simulink model "etr_14b_arch_cleanup"  (R2014b)
settings: Solver=FixedStepDiscrete  SolverMode=SingleTasking  StartTime=0.0  StopTime=inf  FixedStep=balancer_ts  RelTol=1e-3
undefined symbols (not defined in the file): a_d, a_r, balancerStates_Bus0, Batt, battery_gain, battery_offset, cmd_max, current_mode_status, current_task_operation_status, exec_period, Init_Bus0, k_f, k_i, k_phidot, k_thetadot, lightCalib, phi_des, R, STATE, TRACK_MODE_LIST, ts2, W
libraries: legonxtlib x27, simulink x19, simulink_extras x4, ControllersFcns x3, NXTFcns x1
(part 1 of 4)
settings Model: DataDictionary=mainDict.sldd  ExtModeTrigDuration=2  Creator=mbiesiad  LastModifiedBy=pvinnako
settings ConfigSet: Description=Use this configuration to communicate between two robots. This robot is the master.
settings OptimizationCC: OptimizeModelRefInitCode=on  LifeSpan=1
settings DebuggingCC: SolverPrmCheckMsg=none  ParameterPrecisionLossMsg=none  SignalLabelMismatchMsg=error  NonBusSignalsTreatedAsBus=error
settings HardwareCC: ProdLargestAtomicInteger=Long  ProdLargestAtomicFloat=Float  ProdEndianess=LittleEndian  ProdHWDeviceType=ARM Compatible->ARM 7
settings RTWCC: SystemTargetFile=realtime.tlc  GenerateMakefile=off  TemplateMakefile=realtime.tmf  Description=Run on Target Hardware  RTWVerbose=off  ProcessScript=realtime_make_rtw_hook
settings STFCustomTargetCC: TargetLibSuffix=.a  GenerateSampleERTMain=on  ERTCustomFileBanners=on  SupportNonInlinedSFcns=off  SupportVariableSizeSignals=on  MATLABClassNameForMDSCustomization=Simulink.SoftwareTarget.ERTCustomization  GRTInterface=off  SystemTargetFile=realtime.tlc
settings ERTTargetCC: GenerateSampleERTMain=on  ParMdlRefBuildCompliant=off  CompOptLevelCompliant=off  ConcurrentExecutionCompliant=off  CombineOutputUpdateFcns=off  ERTFirstTimeCompliant=off  SupportContinuousTime=on  SupportVariableSizeSignals=on  ModelStepFunctionPrototypeControlCompliant=off  CPPClassGenCompliant=off  ExtModeTransport=1  ExtModeMexFile=ext_serial_win32_comm_no_acks_rtt_byteswap  ExtModeMexArgs=0 1 9600  InlinedParameterPlacement=NonHierarchical  ERTSrcFileBannerTemplate=realtime_code_template.cgt  ERTHdrFileBannerTemplate=realtime_code_template.cgt  ERTDataSrcFileTemplate=realtime_code_template.cgt  ERTDataHdrFileTemplate=realtime_code_template.cgt  ERTCustomFileTemplate=realtime_file_process.tlc

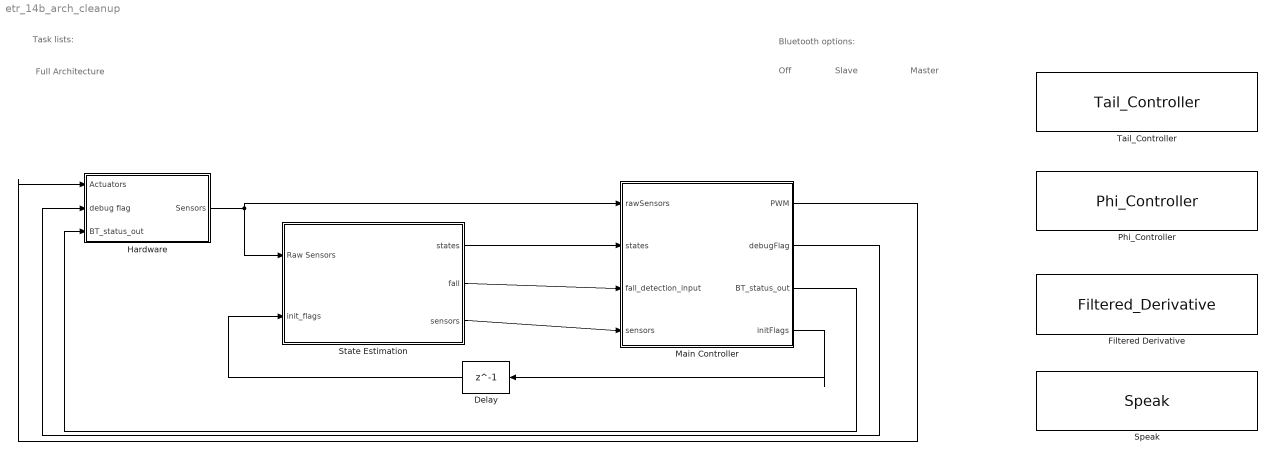
== system etr_14b_arch_cleanup ==
  note: Task lists:
  note: Bluetooth options:
  note: Slave
  note: Master
  note: Off
  note: Full Architecture
  Delay : Delay  DelayLength=1
  Filtered Derivative : ControllersFcns/Filtered_Derivative
  Hardware : Subsystem  VariantControl=Variant1
  Main Controller : Stateflow chart  TreatAsAtomicUnit=on
  Phi_Controller : ControllersFcns/Phi_Controller
  Speak : NXTFcns/Speak
  State Estimation : Subsystem
  Tail_Controller : ControllersFcns/Tail_Controller
  wires:
  State Estimation/2(fall) -> Main Controller/3(fall_detection_input)
  State Estimation/3(sensors) -> Main Controller/4(sensors)
  Hardware/1(Sensors) -> Main Controller/1(rawSensors), State Estimation/1(Raw Sensors)
  Main Controller/4(initFlags) -> Delay/1
  State Estimation/1(states) -> Main Controller/2(states)
  Delay/1 -> State Estimation/2(init_flags)
  Main Controller/2(debugFlag) -> Hardware/2(debug flag)
  Main Controller/1(PWM) -> Hardware/1(Actuators)
  Main Controller/3(BT_status_out) -> Hardware/3(BT_status_out)

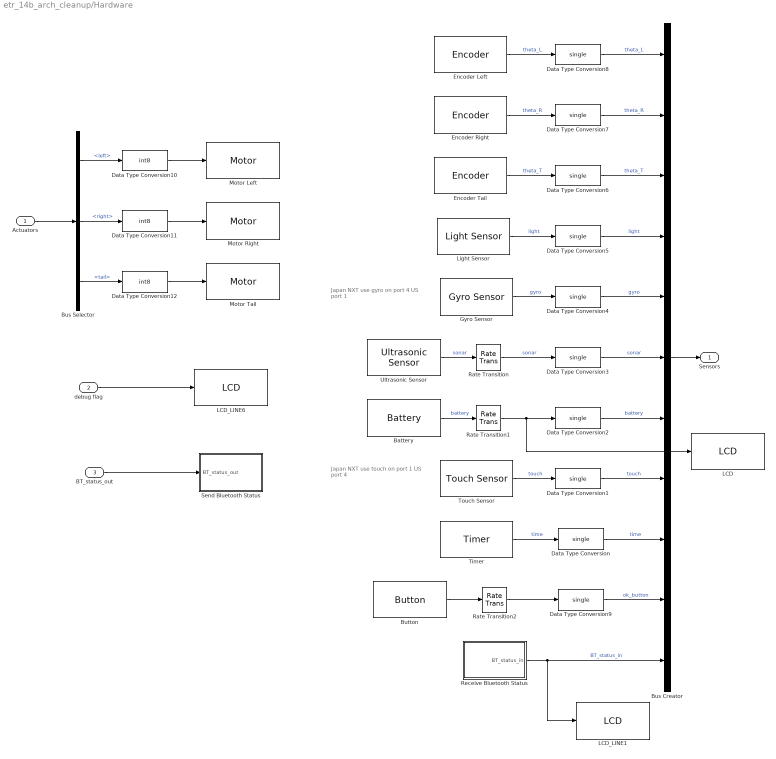
== system etr_14b_arch_cleanup/Hardware ==
  note: Japan NXT use gyro on port 4
      | US port 1
  note: Japan NXT use touch  on port 1
      | US port 4
  Actuators : Inport
  debug flag : Inport  Port=2
  BT_status_out : Inport  Port=3
  Battery : legonxtlib/Battery  sampleTime=.1
  Bus Creator : BusCreator  Inputs=11
  Bus Selector : BusSelector  OutputSignals=left,right,tail
  Button : legonxtlib/Button  buttonType=Middle orange  sampleTime=0.1
  Data Type Conversion{,1..9} (10 alike) : DataTypeConversion  OutDataTypeStr=single
  Data Type Conversion10 : DataTypeConversion  OutDataTypeStr=int8  SaturateOnIntegerOverflow=on
  Data Type Conversion11 : DataTypeConversion  OutDataTypeStr=int8  SaturateOnIntegerOverflow=on
  Data Type Conversion12 : DataTypeConversion  OutDataTypeStr=int8  SaturateOnIntegerOverflow=on
  Encoder Left : legonxtlib/Encoder  portNumber=C  opMode=No reset  sampleTime=0.004
  Encoder Right : legonxtlib/Encoder  portNumber=B  opMode=No reset  sampleTime=0.004
  Encoder Tail : legonxtlib/Encoder  portNumber=A  opMode=No reset  sampleTime=0.004
  Gyro Sensor : legonxtlib/Gyro Sensor  portNumber=1  outputMode=Raw A/D (0 - 1023)  offset=599  sampleTime=0.004
  LCD : legonxtlib/LCD  slcdStr=Batt:  slcdLine=3  slcdFormat=Decimal
  LCD_LINE1 : legonxtlib/LCD  slcdStr=BTSTAT  slcdLine=2  slcdFormat=Decimal
  LCD_LINE6 : legonxtlib/LCD  slcdStr=STATE:  slcdLine=1  slcdFormat=Decimal
  Light Sensor : legonxtlib/Light Sensor  portNumber=3  outputMode=Raw A/D (1023 - 0)  lightOn=on  sampleTime=0.004
  Motor Left : legonxtlib/Motor  sportNumber=C  sstopAction=Brake
  Motor Right : legonxtlib/Motor  sportNumber=B  sstopAction=Brake
  Motor Tail : legonxtlib/Motor  sportNumber=A  sstopAction=Brake
  Rate Transition : RateTransition  OutPortSampleTime=0.004
  Rate Transition1 : RateTransition  OutPortSampleTime=0.004
  Rate Transition2 : RateTransition  OutPortSampleTime=0.004
  Receive Bluetooth Status : Subsystem  Variant=on  OverrideUsingVariant=BluetoothOFF
  Send Bluetooth Status : Subsystem  Variant=on  OverrideUsingVariant=BluetoothOFF
  Timer : legonxtlib/Timer  sampleTime=0.004
  Touch Sensor : legonxtlib/Touch Sensor  portNumber=4  sampleTime=0.004
  Ultrasonic Sensor : legonxtlib/Ultrasonic Sensor  PortNumber=2  sampleTime=0.02
  Sensors : Outport
  wires:
  Receive Bluetooth Status/1(BT_status_in) -> LCD_LINE1/1, Bus Creator/11  "BT_status_in"
  debug flag/1 -> LCD_LINE6/1
  Data Type Conversion9/1 -> Bus Creator/10  "ok_button"
  Rate Transition2/1 -> Data Type Conversion9/1
  Button/1 -> Rate Transition2/1
  Rate Transition1/1 -> LCD/1, Data Type Conversion2/1
  Data Type Conversion8/1 -> Bus Creator/1  "theta_L"
  Data Type Conversion7/1 -> Bus Creator/2  "theta_R"
  Data Type Conversion6/1 -> Bus Creator/3  "theta_T"
  Data Type Conversion5/1 -> Bus Creator/4  "light"
  Data Type Conversion4/1 -> Bus Creator/5  "gyro"
  Data Type Conversion3/1 -> Bus Creator/6  "sonar"
  Data Type Conversion2/1 -> Bus Creator/7  "battery"
  Data Type Conversion1/1 -> Bus Creator/8  "touch"
  Data Type Conversion/1 -> Bus Creator/9  "time"
  Rate Transition/1 -> Data Type Conversion3/1  "sonar"
  Ultrasonic Sensor/1 -> Rate Transition/1  "sonar"
  Bus Selector/3 -> Data Type Conversion12/1  "<tail>"
  Encoder Tail/1 -> Data Type Conversion6/1  "theta_T"
  Light Sensor/1 -> Data Type Conversion5/1  "light"
  Bus Selector/2 -> Data Type Conversion11/1  "<right>"
  Bus Selector/1 -> Data Type Conversion10/1  "<left>"
  Touch Sensor/1 -> Data Type Conversion1/1  "touch"
  Bus Creator/1 -> Sensors/1
  Battery/1 -> Rate Transition1/1  "battery"
  Gyro Sensor/1 -> Data Type Conversion4/1  "gyro"
  Encoder Right/1 -> Data Type Conversion7/1  "theta_R"
  Encoder Left/1 -> Data Type Conversion8/1  "theta_L"
  Timer/1 -> Data Type Conversion/1  "time"
  Actuators/1 -> Bus Selector/1
  Data Type Conversion10/1 -> Motor Left/1
  Data Type Conversion11/1 -> Motor Right/1
  Data Type Conversion12/1 -> Motor Tail/1
  BT_status_out/1 -> Send Bluetooth Status/1(BT_status_out)

== system etr_14b_arch_cleanup/Main Controller/normal_operation_modes.gyro_calibration_mode ==
  sensors : Inport
  " Demux " : Demux  Outputs=1
  " SFunction " : S-Function  Tag=Stateflow S-Function etr_14b_arch_cleanup 10  FunctionName=sf_sfun  PortCounts=[1 4]  EnableBusSupport=off
  gyro_calibration_mode.GyroCalibration.Speak : Subsystem  Commented=on
      settings: UndoDeleteFcn=Stateflow.SLINSF.SimulinkMan.restorePreDeleteFcn  PreDeleteFcn=Stateflow.SLINSF.SimulinkMan.removePreDeleteFcn
  debugFlag : Outport
  initFlags : Outport  Port=2
  PWM : Outport  Port=3
  wires:
  sensors/1 -> " SFunction "/1
  " SFunction "/2 -> debugFlag/1  "debugFlag"
  " SFunction "/3 -> initFlags/1  "initFlags"
  " SFunction "/4 -> PWM/1  "PWM"
  " Demux "/1 -> gyro_calibration_mode.GyroCalibration.Speak/Trigger
  " SFunction "/1 -> " Demux "/1

== system etr_14b_arch_cleanup/Main Controller/normal_operation_modes.light_calibration_up ==
  sensors : Inport
  " Demux " : Demux  Outputs=1
  " SFunction " : S-Function  Tag=Stateflow S-Function etr_14b_arch_cleanup 7  FunctionName=sf_sfun  PortCounts=[1 4]  EnableBusSupport=off
  Speak : Subsystem  Commented=on
      settings: UndoDeleteFcn=Stateflow.SLINSF.SimulinkMan.restorePreDeleteFcn  PreDeleteFcn=Stateflow.SLINSF.SimulinkMan.removePreDeleteFcn
  debugFlag : Outport
  PWM : Outport  Port=2
  initFlags : Outport  Port=3
  wires:
  sensors/1 -> " SFunction "/1
  " SFunction "/2 -> debugFlag/1  "debugFlag"
  " SFunction "/3 -> PWM/1  "PWM"
  " SFunction "/4 -> initFlags/1  "initFlags"
  " Demux "/1 -> Speak/Trigger
  " SFunction "/1 -> " Demux "/1

== system etr_14b_arch_cleanup/Main Controller/normal_operation_modes.light_calibration_up_flashing ==
  sensors : Inport
  " Demux " : Demux
  " SFunction " : S-Function  Tag=Stateflow S-Function etr_14b_arch_cleanup 8  FunctionName=sf_sfun  PortCounts=[2 4]  EnableBusSupport=off
  LightSensorCalibFlashing.Speak : Subsystem  Commented=on
      settings: UndoDeleteFcn=Stateflow.SLINSF.SimulinkMan.restorePreDeleteFcn  PreDeleteFcn=Stateflow.SLINSF.SimulinkMan.removePreDeleteFcn
  LightSensorCalibFlashing.processLight : Subsystem
      settings: UndoDeleteFcn=Stateflow.SLINSF.SimulinkMan.restorePreDeleteFcn  PreDeleteFcn=Stateflow.SLINSF.SimulinkMan.removePreDeleteFcn
  LightSensorCalibFlashing.showCalib : Subsystem  Commented=on
      settings: UndoDeleteFcn=Stateflow.SLINSF.SimulinkMan.restorePreDeleteFcn  PreDeleteFcn=Stateflow.SLINSF.SimulinkMan.removePreDeleteFcn
  LightSensorCalibFlashing.turnLightOn : Subsystem
      settings: UndoDeleteFcn=Stateflow.SLINSF.SimulinkMan.restorePreDeleteFcn  PreDeleteFcn=Stateflow.SLINSF.SimulinkMan.removePreDeleteFcn
  debugFlag : Outport
  wires:
  sensors/1 -> " SFunction "/1
  " SFunction "/2 -> debugFlag/1  "debugFlag"
  " SFunction "/3 -> LightSensorCalibFlashing.showCalib/1(lightCalib)
  " Demux "/1 -> LightSensorCalibFlashing.showCalib/Trigger
  " Demux "/2 -> LightSensorCalibFlashing.Speak/Trigger
  " Demux "/3 -> LightSensorCalibFlashing.turnLightOn/Trigger
  " SFunction "/4 -> LightSensorCalibFlashing.processLight/1(rawLight)
  LightSensorCalibFlashing.processLight/1(filteredLight) -> " SFunction "/2
  " Demux "/4 -> LightSensorCalibFlashing.processLight/Trigger
  " SFunction "/1 -> " Demux "/1

== system etr_14b_arch_cleanup/Main Controller/normal_operation_modes.light_calibration_up_flashing_on_map ==
  sensors : Inport
  " Demux " : Demux  Outputs=3
  " SFunction " : S-Function  Tag=Stateflow S-Function etr_14b_arch_cleanup 9  FunctionName=sf_sfun  PortCounts=[2 3]  EnableBusSupport=off
  LightSensorCalibFlashing.Speak : Subsystem  Commented=on
      settings: UndoDeleteFcn=Stateflow.SLINSF.SimulinkMan.restorePreDeleteFcn  PreDeleteFcn=Stateflow.SLINSF.SimulinkMan.removePreDeleteFcn
  LightSensorCalibFlashing.processLight : Subsystem
      settings: UndoDeleteFcn=Stateflow.SLINSF.SimulinkMan.restorePreDeleteFcn  PreDeleteFcn=Stateflow.SLINSF.SimulinkMan.removePreDeleteFcn
  LightSensorCalibFlashing.turnLightOn : Subsystem
      settings: UndoDeleteFcn=Stateflow.SLINSF.SimulinkMan.restorePreDeleteFcn  PreDeleteFcn=Stateflow.SLINSF.SimulinkMan.removePreDeleteFcn
  debugFlag : Outport
  wires:
  sensors/1 -> " SFunction "/1
  " SFunction "/2 -> debugFlag/1  "debugFlag"
  " Demux "/1 -> LightSensorCalibFlashing.Speak/Trigger
  " Demux "/2 -> LightSensorCalibFlashing.turnLightOn/Trigger
  " SFunction "/3 -> LightSensorCalibFlashing.processLight/1(rawLight)
  LightSensorCalibFlashing.processLight/1(filteredLight) -> " SFunction "/2
  " Demux "/3 -> LightSensorCalibFlashing.processLight/Trigger
  " SFunction "/1 -> " Demux "/1

== system etr_14b_arch_cleanup/Main Controller/normal_operation_modes.line_tracking_after_seesaw ==
  sensors : Inport
  states : Inport  Port=2
  rawSensors : Inport  Port=3
  " Demux " : Demux  Outputs=7
  " SFunction " : S-Function  Tag=Stateflow S-Function etr_14b_arch_cleanup 6  FunctionName=sf_sfun  PortCounts=[13 17]  EnableBusSupport=off
  line_tracking_mode.Speak : Subsystem  Commented=on
      settings: UndoDeleteFcn=Stateflow.SLINSF.SimulinkMan.restorePreDeleteFcn  PreDeleteFcn=Stateflow.SLINSF.SimulinkMan.removePreDeleteFcn
  line_tracking_mode.Track.analyzeEncoders : Subsystem
      settings: UndoDeleteFcn=Stateflow.SLINSF.SimulinkMan.restorePreDeleteFcn  PreDeleteFcn=Stateflow.SLINSF.SimulinkMan.removePreDeleteFcn
  line_tracking_mode.Track.lineTracker : Subsystem
      settings: UndoDeleteFcn=Stateflow.SLINSF.SimulinkMan.restorePreDeleteFcn  PreDeleteFcn=Stateflow.SLINSF.SimulinkMan.removePreDeleteFcn
  line_tracking_mode.Track.processLight : Subsystem
      settings: UndoDeleteFcn=Stateflow.SLINSF.SimulinkMan.restorePreDeleteFcn  PreDeleteFcn=Stateflow.SLINSF.SimulinkMan.removePreDeleteFcn
  line_tracking_mode.balanceControl : Subsystem
      settings: UndoDeleteFcn=Stateflow.SLINSF.SimulinkMan.restorePreDeleteFcn  PreDeleteFcn=Stateflow.SLINSF.SimulinkMan.removePreDeleteFcn
  line_tracking_mode.phiController : Subsystem
      settings: UndoDeleteFcn=Stateflow.SLINSF.SimulinkMan.restorePreDeleteFcn  PreDeleteFcn=Stateflow.SLINSF.SimulinkMan.removePreDeleteFcn
  line_tracking_mode.turnLightOn : Subsystem
      settings: UndoDeleteFcn=Stateflow.SLINSF.SimulinkMan.restorePreDeleteFcn  PreDeleteFcn=Stateflow.SLINSF.SimulinkMan.removePreDeleteFcn
  PWM : Outport
  debugFlag : Outport  Port=2
  initFlags : Outport  Port=3
  wires:
  sensors/1 -> " SFunction "/1
  states/1 -> " SFunction "/2
  rawSensors/1 -> " SFunction "/3
  " SFunction "/2 -> PWM/1  "PWM"
  " SFunction "/3 -> debugFlag/1  "debugFlag"
  " SFunction "/4 -> initFlags/1  "initFlags"
  " SFunction "/5 -> line_tracking_mode.Track.processLight/1(rawLight)
  " SFunction "/6 -> line_tracking_mode.Track.processLight/2(bias)
  " SFunction "/7 -> line_tracking_mode.Track.processLight/3(lightCalib)
  line_tracking_mode.Track.processLight/1(normalizedLight) -> " SFunction "/4
  line_tracking_mode.Track.processLight/2(filteredLight) -> " SFunction "/5
  " Demux "/1 -> line_tracking_mode.Track.processLight/Trigger
  " SFunction "/8 -> line_tracking_mode.Track.analyzeEncoders/1(rawSensors)
  line_tracking_mode.Track.analyzeEncoders/1(AngleCount) -> " SFunction "/6
  line_tracking_mode.Track.analyzeEncoders/2(EncoderReset) -> " SFunction "/7
  line_tracking_mode.Track.analyzeEncoders/3(Angle) -> " SFunction "/8
  line_tracking_mode.Track.analyzeEncoders/4(Distance) -> " SFunction "/9
  " Demux "/2 -> line_tracking_mode.Track.analyzeEncoders/Trigger
  " SFunction "/9 -> line_tracking_mode.Track.lineTracker/1(lightSignal)
  " SFunction "/10 -> line_tracking_mode.Track.lineTracker/2(flagSteering)
  " SFunction "/11 -> line_tracking_mode.Track.lineTracker/3(PID)
  " SFunction "/12 -> line_tracking_mode.Track.lineTracker/4(fwd)
  line_tracking_mode.Track.lineTracker/1(cmd) -> " SFunction "/10
  " Demux "/3 -> line_tracking_mode.Track.lineTracker/Trigger
  " SFunction "/13 -> line_tracking_mode.phiController/1(phi)
  " SFunction "/14 -> line_tracking_mode.phiController/2(desiredPhi)
  " SFunction "/15 -> line_tracking_mode.phiController/3(battery)
  line_tracking_mode.phiController/1(cmd) -> " SFunction "/11
  " Demux "/4 -> line_tracking_mode.phiController/Trigger
  " SFunction "/16 -> line_tracking_mode.balanceControl/1(rawSensors)
  " SFunction "/17 -> line_tracking_mode.balanceControl/2(lineTrackCmd)
  line_tracking_mode.balanceControl/1(leftPWM) -> " SFunction "/12
  line_tracking_mode.balanceControl/2(rightPWM) -> " SFunction "/13
  " Demux "/5 -> line_tracking_mode.balanceControl/Trigger
  " Demux "/6 -> line_tracking_mode.turnLightOn/Trigger
  " Demux "/7 -> line_tracking_mode.Speak/Trigger
  " SFunction "/1 -> " Demux "/1

== system etr_14b_arch_cleanup/Main Controller/normal_operation_modes.line_tracking_mode ==
  sensors : Inport
  states : Inport  Port=2
  rawSensors : Inport  Port=3
  " Demux " : Demux  Outputs=7
  " SFunction " : S-Function  Tag=Stateflow S-Function etr_14b_arch_cleanup 2  FunctionName=sf_sfun  PortCounts=[13 18]  EnableBusSupport=off
  line_tracking_mode.Speak : Subsystem  Commented=on
      settings: UndoDeleteFcn=Stateflow.SLINSF.SimulinkMan.restorePreDeleteFcn  PreDeleteFcn=Stateflow.SLINSF.SimulinkMan.removePreDeleteFcn
  line_tracking_mode.Track.analyzeEncoders : Subsystem
      settings: UndoDeleteFcn=Stateflow.SLINSF.SimulinkMan.restorePreDeleteFcn  PreDeleteFcn=Stateflow.SLINSF.SimulinkMan.removePreDeleteFcn
  line_tracking_mode.Track.lineTracker : Subsystem
      settings: UndoDeleteFcn=Stateflow.SLINSF.SimulinkMan.restorePreDeleteFcn  PreDeleteFcn=Stateflow.SLINSF.SimulinkMan.removePreDeleteFcn
  line_tracking_mode.Track.processLight : Subsystem
      settings: UndoDeleteFcn=Stateflow.SLINSF.SimulinkMan.restorePreDeleteFcn  PreDeleteFcn=Stateflow.SLINSF.SimulinkMan.removePreDeleteFcn
  line_tracking_mode.balanceControl : Subsystem
      settings: UndoDeleteFcn=Stateflow.SLINSF.SimulinkMan.restorePreDeleteFcn  PreDeleteFcn=Stateflow.SLINSF.SimulinkMan.removePreDeleteFcn
  line_tracking_mode.phiController : Subsystem
      settings: UndoDeleteFcn=Stateflow.SLINSF.SimulinkMan.restorePreDeleteFcn  PreDeleteFcn=Stateflow.SLINSF.SimulinkMan.removePreDeleteFcn
  line_tracking_mode.turnLightOn : Subsystem
      settings: UndoDeleteFcn=Stateflow.SLINSF.SimulinkMan.restorePreDeleteFcn  PreDeleteFcn=Stateflow.SLINSF.SimulinkMan.removePreDeleteFcn
  PWM : Outport
  debugFlag : Outport  Port=2
  wires:
  sensors/1 -> " SFunction "/1
  states/1 -> " SFunction "/2
  rawSensors/1 -> " SFunction "/3
  " SFunction "/2 -> PWM/1  "PWM"
  " SFunction "/3 -> debugFlag/1  "debugFlag"
  " SFunction "/4 -> line_tracking_mode.Track.processLight/1(rawLight)
  " SFunction "/5 -> line_tracking_mode.Track.processLight/2(bias)
  " SFunction "/6 -> line_tracking_mode.Track.processLight/3(minLight)
  " SFunction "/7 -> line_tracking_mode.Track.processLight/4(maxLight)
  line_tracking_mode.Track.processLight/1(normalizedLight) -> " SFunction "/4
  line_tracking_mode.Track.processLight/2(filteredLight) -> " SFunction "/5
  " Demux "/1 -> line_tracking_mode.Track.processLight/Trigger
  " SFunction "/8 -> line_tracking_mode.Track.analyzeEncoders/1(rawSensors)
  line_tracking_mode.Track.analyzeEncoders/1(AngleCount) -> " SFunction "/6
  line_tracking_mode.Track.analyzeEncoders/2(EncoderReset) -> " SFunction "/7
  line_tracking_mode.Track.analyzeEncoders/3(Angle) -> " SFunction "/8
  line_tracking_mode.Track.analyzeEncoders/4(Distance) -> " SFunction "/9
  " Demux "/2 -> line_tracking_mode.Track.analyzeEncoders/Trigger
  " SFunction "/9 -> line_tracking_mode.Track.lineTracker/1(lightSignal)
  " SFunction "/10 -> line_tracking_mode.Track.lineTracker/2(flagSteering)
  " SFunction "/11 -> line_tracking_mode.Track.lineTracker/3(PID)
  " SFunction "/12 -> line_tracking_mode.Track.lineTracker/4(fwd)
  line_tracking_mode.Track.lineTracker/1(cmd) -> " SFunction "/10
  " Demux "/3 -> line_tracking_mode.Track.lineTracker/Trigger
  " SFunction "/13 -> line_tracking_mode.phiController/1(phi)
  " SFunction "/14 -> line_tracking_mode.phiController/2(desiredPhi)
  " SFunction "/15 -> line_tracking_mode.phiController/3(battery)
  line_tracking_mode.phiController/1(cmd) -> " SFunction "/11
  " Demux "/4 -> line_tracking_mode.phiController/Trigger
  " SFunction "/16 -> line_tracking_mode.balanceControl/1(rawSensors)
  " SFunction "/17 -> line_tracking_mode.balanceControl/2(lineTrackCmd)
  " SFunction "/18 -> line_tracking_mode.balanceControl/3(gyroTrick)
  line_tracking_mode.balanceControl/1(leftPWM) -> " SFunction "/12
  line_tracking_mode.balanceControl/2(rightPWM) -> " SFunction "/13
  " Demux "/5 -> line_tracking_mode.balanceControl/Trigger
  " Demux "/6 -> line_tracking_mode.turnLightOn/Trigger
  " Demux "/7 -> line_tracking_mode.Speak/Trigger
  " SFunction "/1 -> " Demux "/1

== system etr_14b_arch_cleanup/State Estimation ==
  Raw Sensors : Inport
  init_flags : Inport  Port=2
  Bus Selector1 : BusSelector  OutputSignals=tail,gyroInit,gyroReset,theta,fall
  Data Type Conversion Unit Conversion Tail Initialization : Subsystem
  Fall Detection : Subsystem
  Gyro Processing : Subsystem
  StateEstimation : Subsystem
  states : Outport
  fall : Outport  Port=2
  sensors : Outport  Port=3
  wires:
  Bus Selector1/3 -> Gyro Processing/3(gyroReset)  "<gyroReset>"
  Bus Selector1/4 -> StateEstimation/4(init theta)  "<theta>"
  Bus Selector1/1 -> Data Type Conversion Unit Conversion Tail Initialization/2(init_tail)  "<tail>"
  Bus Selector1/2 -> Gyro Processing/2(gyroInit)  "<gyroInit>"
  init_flags/1 -> Bus Selector1/1
  StateEstimation/1(states) -> states/1  "states"
  Data Type Conversion Unit Conversion Tail Initialization/1(y) -> Gyro Processing/1(sensors), sensors/1, StateEstimation/1(Sensors)
  Raw Sensors/1 -> Data Type Conversion Unit Conversion Tail Initialization/1(u)
  Gyro Processing/1(psi) -> StateEstimation/2(psi)
  Gyro Processing/2(psi_dot) -> StateEstimation/3(psi_dot)
  Gyro Processing/3(psi filtered) -> Fall Detection/1(gyro)
  Bus Selector1/5 -> Fall Detection/2(reset)  "<fall>"
  Fall Detection/1(fall_detected) -> fall/1

== system etr_14b_arch_cleanup/Hardware/Receive Bluetooth Status ==
  note: 1) Only subsystems can be added as variant choices at this level
      | 2) Blocks cannot be connected at this level as connectivity is
      | automatically determined at simulation, based on the active variant
  BluetoothOFF : Subsystem  VariantControl=BluetoothOFF
  BluetoothONMario : Subsystem  VariantControl=BluetoothONMario
  BluetoothONPrincess : Subsystem  VariantControl=BluetoothONPrincess
  BT_status_in : Outport

== system etr_14b_arch_cleanup/Hardware/Send Bluetooth Status ==
  note: 1) Only subsystems can be added as variant choices at this level
      | 2) Blocks cannot be connected at this level as connectivity is
      | automatically determined at simulation, based on the active variant
  BT_status_out : Inport
  BluetoothOFF : Subsystem  VariantControl=BluetoothOFF
  BluetoothONMario : Subsystem  VariantControl=BluetoothONMario
  BluetoothONPrincess : Subsystem  VariantControl=BluetoothONPrincess

== system etr_14b_arch_cleanup/Main Controller/normal_operation_modes.gyro_calibration_mode/gyro_calibration_mode.GyroCalibration.Speak ==
  f : TriggerPort  TriggerType=function-call
      settings: CopyFcn=Stateflow.SLINSF.SimulinkMan.removeBlockPreDeleteFcn  PreDeleteFcn=Stateflow.SLINSF.SimulinkMan.unsafePredeleteFcn
  Constant : Constant  Value=50
  Speaker : legonxtlib/Speaker  sinputMode=Volume only  sspeakerFreq=800  sspeakerVolume=50  sspeakerDuration=100
  wires:
  Constant/1 -> Speaker/1

== system etr_14b_arch_cleanup/Main Controller/normal_operation_modes.light_calibration_up/Speak ==
  f : TriggerPort  TriggerType=function-call
      settings: CopyFcn=Stateflow.SLINSF.SimulinkMan.removeBlockPreDeleteFcn  PreDeleteFcn=Stateflow.SLINSF.SimulinkMan.unsafePredeleteFcn
  Constant : Constant  Value=50
  Speaker : legonxtlib/Speaker  sinputMode=Volume only  sspeakerFreq=800  sspeakerVolume=50  sspeakerDuration=100
  wires:
  Constant/1 -> Speaker/1

== system etr_14b_arch_cleanup/Main Controller/normal_operation_modes.light_calibration_up_flashing/LightSensorCalibFlashing.Speak ==
  f : TriggerPort  TriggerType=function-call
      settings: CopyFcn=Stateflow.SLINSF.SimulinkMan.removeBlockPreDeleteFcn  PreDeleteFcn=Stateflow.SLINSF.SimulinkMan.unsafePredeleteFcn
  Constant : Constant  Value=50
  Speaker : legonxtlib/Speaker  sinputMode=Volume only  sspeakerFreq=800  sspeakerVolume=50  sspeakerDuration=100
  wires:
  Constant/1 -> Speaker/1

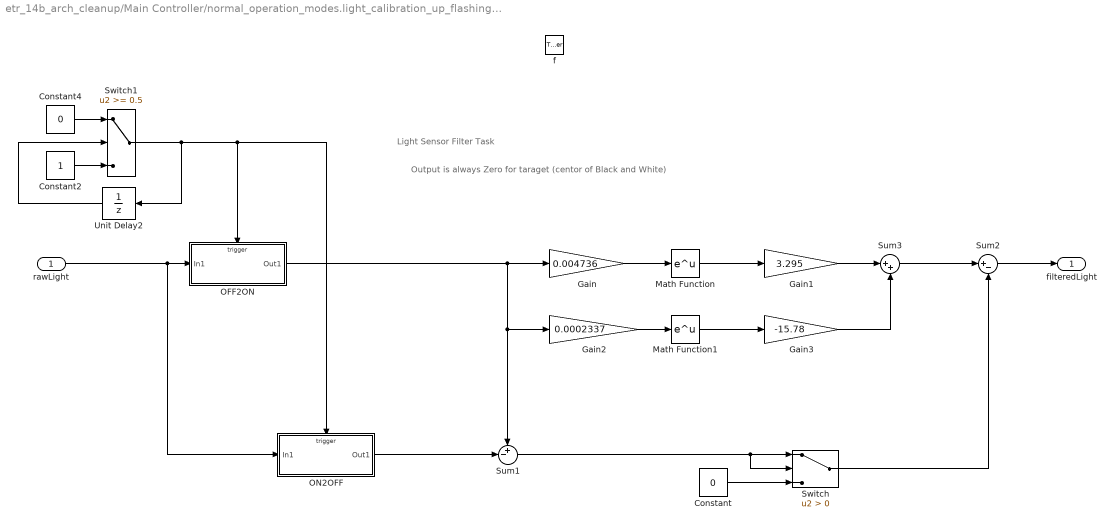
== system etr_14b_arch_cleanup/Main Controller/normal_operation_modes.light_calibration_up_flashing/LightSensorCalibFlashing.processLight ==
  note: Output is always Zero for taraget (centor of Black and White)
  note: Light Sensor Filter Task
  rawLight : Inport  OutDataTypeStr=single  PortDimensions=1
  f : TriggerPort  TriggerType=function-call
      settings: CopyFcn=Stateflow.SLINSF.SimulinkMan.removeBlockPreDeleteFcn  PreDeleteFcn=Stateflow.SLINSF.SimulinkMan.unsafePredeleteFcn
  Constant : Constant  Value=0  OutDataTypeStr=single  SampleTime=-1
  Constant2 : Constant  OutDataTypeStr=uint8
  Constant4 : Constant  Value=0  OutDataTypeStr=uint8
  Gain : Gain  Gain=0.004736
  Gain1 : Gain  Gain=3.295
  Gain2 : Gain  Gain=0.0002337
  Gain3 : Gain  Gain=-15.78
  Math Function : Math  SaturateOnIntegerOverflow=on
  Math Function1 : Math  SaturateOnIntegerOverflow=on
  OFF2ON : Subsystem  TreatAsAtomicUnit=on
  ON2OFF : Subsystem  TreatAsAtomicUnit=on
  Sum1 : Sum  Inputs=+-|
  Sum2 : Sum  Inputs=|+-
  Sum3 : Sum  Inputs=|++
  Switch : Switch  Criteria=u2 > Threshold  RndMeth=Simplest
  Switch1 : Switch  Threshold=0.5
  Unit Delay2 : UnitDelay  SampleTime=-1
  filteredLight : Outport  OutDataTypeStr=single  PortDimensions=1  InitialOutput=0
  wires:
  Sum2/1 -> filteredLight/1
  Switch/1 -> Sum2/2
  Sum3/1 -> Sum2/1
  Gain3/1 -> Sum3/2
  Gain1/1 -> Sum3/1
  Math Function1/1 -> Gain3/1
  Gain2/1 -> Math Function1/1
  Sum1/1 -> Switch/2, Switch/1
  Constant/1 -> Switch/3
  Math Function/1 -> Gain1/1
  Gain/1 -> Math Function/1
  OFF2ON/1(Out1) -> Gain2/1, Sum1/1, Gain/1
  ON2OFF/1(Out1) -> Sum1/2
  Unit Delay2/1 -> Switch1/2
  Constant4/1 -> Switch1/1
  Constant2/1 -> Switch1/3
  Switch1/1 -> Unit Delay2/1, OFF2ON/Trigger, ON2OFF/Trigger
  rawLight/1 -> ON2OFF/1(In1), OFF2ON/1(In1)

== system etr_14b_arch_cleanup/Main Controller/normal_operation_modes.light_calibration_up_flashing/LightSensorCalibFlashing.showCalib ==
  lightCalib : Inport  OutDataTypeStr=Bus: Light_Bus  PortDimensions=1
  f : TriggerPort  TriggerType=function-call
      settings: CopyFcn=Stateflow.SLINSF.SimulinkMan.removeBlockPreDeleteFcn  PreDeleteFcn=Stateflow.SLINSF.SimulinkMan.unsafePredeleteFcn
  Bus Selector : BusSelector  OutputSignals=flashingWhite,flashingBlack
  wires:
  lightCalib/1 -> Bus Selector/1
  Bus Selector/1 -> ?  "<flashingWhite>"
  Bus Selector/2 -> ?  "<flashingBlack>"

== system etr_14b_arch_cleanup/Main Controller/normal_operation_modes.light_calibration_up_flashing/LightSensorCalibFlashing.turnLightOn ==
  f : TriggerPort  TriggerType=function-call
      settings: CopyFcn=Stateflow.SLINSF.SimulinkMan.removeBlockPreDeleteFcn  PreDeleteFcn=Stateflow.SLINSF.SimulinkMan.unsafePredeleteFcn
  Light Sensor Switch ON : S-Function  FunctionName=sfun_light_sw  Parameters=-1,ip,sw  EnableBusSupport=off  mask(Light Sensor ON/OFF Switch){ip=S3, sw=ON}
      mask prompts: ip "port:"; sw "switch"
      mask help: LEGO Mindstorms NXT Light Sensor switch.
      mask init:
      | [data, map]=imread('LIGHT_SENSOR.gif');
      | pic=ind2rgb(data,map);
      mask TypeOptions ip: S1 | S2 | S3 | S4
      mask TypeOptions sw: ON | OFF
      mask Display:
      | image(pic)
      | color('red')
      | fprintf('%s, %s',ip,sw)

== system etr_14b_arch_cleanup/Main Controller/normal_operation_modes.light_calibration_up_flashing_on_map/LightSensorCalibFlashing.Speak ==
  f : TriggerPort  TriggerType=function-call
      settings: CopyFcn=Stateflow.SLINSF.SimulinkMan.removeBlockPreDeleteFcn  PreDeleteFcn=Stateflow.SLINSF.SimulinkMan.unsafePredeleteFcn
  Constant : Constant  Value=50
  Speaker : legonxtlib/Speaker  sinputMode=Volume only  sspeakerFreq=800  sspeakerVolume=50  sspeakerDuration=100
  wires:
  Constant/1 -> Speaker/1

== system etr_14b_arch_cleanup/Main Controller/normal_operation_modes.light_calibration_up_flashing_on_map/LightSensorCalibFlashing.processLight ==
  note: Output is always Zero for taraget (centor of Black and White)
  note: Light Sensor Filter Task
  rawLight : Inport  OutDataTypeStr=single  PortDimensions=1
  f : TriggerPort  TriggerType=function-call
      settings: CopyFcn=Stateflow.SLINSF.SimulinkMan.removeBlockPreDeleteFcn  PreDeleteFcn=Stateflow.SLINSF.SimulinkMan.unsafePredeleteFcn
  Constant : Constant  Value=0  OutDataTypeStr=single  SampleTime=-1
  Constant2 : Constant  OutDataTypeStr=uint8
  Constant4 : Constant  Value=0  OutDataTypeStr=uint8
  Gain : Gain  Gain=0.004736
  Gain1 : Gain  Gain=3.295
  Gain2 : Gain  Gain=0.0002337
  Gain3 : Gain  Gain=-15.78
  Math Function : Math  SaturateOnIntegerOverflow=on
  Math Function1 : Math  SaturateOnIntegerOverflow=on
  OFF2ON : Subsystem  TreatAsAtomicUnit=on
  ON2OFF : Subsystem  TreatAsAtomicUnit=on
  Sum1 : Sum  Inputs=+-|
  Sum2 : Sum  Inputs=|+-
  Sum3 : Sum  Inputs=|++
  Switch : Switch  Criteria=u2 > Threshold  RndMeth=Simplest
  Switch1 : Switch  Threshold=0.5
  Unit Delay2 : UnitDelay  SampleTime=-1
  filteredLight : Outport  OutDataTypeStr=single  PortDimensions=1  InitialOutput=0
  wires:
  Sum2/1 -> filteredLight/1
  Switch/1 -> Sum2/2
  Sum3/1 -> Sum2/1
  Gain3/1 -> Sum3/2
  Gain1/1 -> Sum3/1
  Math Function1/1 -> Gain3/1
  Gain2/1 -> Math Function1/1
  Sum1/1 -> Switch/2, Switch/1
  Constant/1 -> Switch/3
  Math Function/1 -> Gain1/1
  Gain/1 -> Math Function/1
  OFF2ON/1(Out1) -> Gain2/1, Sum1/1, Gain/1
  ON2OFF/1(Out1) -> Sum1/2
  Unit Delay2/1 -> Switch1/2
  Constant4/1 -> Switch1/1
  Constant2/1 -> Switch1/3
  Switch1/1 -> Unit Delay2/1, OFF2ON/Trigger, ON2OFF/Trigger
  rawLight/1 -> ON2OFF/1(In1), OFF2ON/1(In1)

== system etr_14b_arch_cleanup/Main Controller/normal_operation_modes.light_calibration_up_flashing_on_map/LightSensorCalibFlashing.turnLightOn ==
  f : TriggerPort  TriggerType=function-call
      settings: CopyFcn=Stateflow.SLINSF.SimulinkMan.removeBlockPreDeleteFcn  PreDeleteFcn=Stateflow.SLINSF.SimulinkMan.unsafePredeleteFcn
  Light Sensor Switch ON : S-Function  FunctionName=sfun_light_sw  Parameters=-1,ip,sw  EnableBusSupport=off  mask(Light Sensor ON/OFF Switch){ip=S3, sw=ON}
      mask prompts: ip "port:"; sw "switch"
      mask help: LEGO Mindstorms NXT Light Sensor switch.
      mask init:
      | [data, map]=imread('LIGHT_SENSOR.gif');
      | pic=ind2rgb(data,map);
      mask TypeOptions ip: S1 | S2 | S3 | S4
      mask TypeOptions sw: ON | OFF
      mask Display:
      | image(pic)
      | color('red')
      | fprintf('%s, %s',ip,sw)

== system etr_14b_arch_cleanup/Main Controller/normal_operation_modes.line_tracking_after_seesaw/line_tracking_mode.Speak ==
  f : TriggerPort  TriggerType=function-call
      settings: CopyFcn=Stateflow.SLINSF.SimulinkMan.removeBlockPreDeleteFcn  PreDeleteFcn=Stateflow.SLINSF.SimulinkMan.unsafePredeleteFcn
  Constant : Constant  Value=50
  Speaker : legonxtlib/Speaker  sinputMode=Volume only  sspeakerFreq=800  sspeakerVolume=50  sspeakerDuration=100
  wires:
  Constant/1 -> Speaker/1

== system etr_14b_arch_cleanup/Main Controller/normal_operation_modes.line_tracking_after_seesaw/line_tracking_mode.Track.analyzeEncoders ==
  rawSensors : Inport  OutDataTypeStr=Bus: Sensors_Bus  PortDimensions=1
  f : TriggerPort  TriggerType=function-call
      settings: CopyFcn=Stateflow.SLINSF.SimulinkMan.removeBlockPreDeleteFcn  PreDeleteFcn=Stateflow.SLINSF.SimulinkMan.unsafePredeleteFcn
  AngleCounter : Subsystem
  Bus Creator : BusCreator  Inputs=2
  Bus Selector : BusSelector  OutputSignals=theta_R,theta_L
  Constant : Constant  Value=0
  Memory : Memory  X0=1  InheritSampleTime=on
  Signal Conversion : SignalConversion
  Signal Conversion1 : SignalConversion
  Store x0 : Subsystem  TreatAsAtomicUnit=on
  Sum : Sum  Inputs=-+|
  Sum1 : Sum  Inputs=-+|
  AngleCount : Outport  OutDataTypeStr=uint8  PortDimensions=1  InitialOutput=0
  EncoderReset : Outport  Port=2  OutDataTypeStr=single  PortDimensions=1  InitialOutput=0
  Angle : Outport  Port=3  OutDataTypeStr=single  PortDimensions=1  InitialOutput=0
  Distance : Outport  Port=4  OutDataTypeStr=single  PortDimensions=1  InitialOutput=0
  wires:
  rawSensors/1 -> Bus Selector/1
  Bus Creator/1 -> AngleCounter/1(EC)
  Bus Selector/1 -> Store x0/1(In1), Sum/2  "<theta_R>"
  Bus Selector/2 -> Sum1/2, Store x0/2(In2)  "<theta_L>"
  Signal Conversion/1 -> Bus Creator/1  "R"
  Signal Conversion1/1 -> Bus Creator/2  "L"
  AngleCounter/1(AngleCount) -> AngleCount/1
  AngleCounter/2(EncoderReseted) -> EncoderReset/1
  AngleCounter/3(Angle) -> Angle/1
  AngleCounter/4(Distance) -> Distance/1
  Constant/1 -> Memory/1
  Memory/1 -> Store x0/Enable
  Sum/1 -> Signal Conversion/1
  Sum1/1 -> Signal Conversion1/1
  Store x0/2(Out2) -> Sum1/1
  Store x0/1(Out1) -> Sum/1

== system etr_14b_arch_cleanup/Main Controller/normal_operation_modes.line_tracking_after_seesaw/line_tracking_mode.Track.lineTracker ==
  lightSignal : Inport  OutDataTypeStr=single  PortDimensions=1
  flagSteering : Inport  Port=2  OutDataTypeStr=single  PortDimensions=1
  PID : Inport  Port=3  OutDataTypeStr=single  PortDimensions=5
  fwd : Inport  Port=4  OutDataTypeStr=single  PortDimensions=1
  f : TriggerPort  TriggerType=function-call
      settings: CopyFcn=Stateflow.SLINSF.SimulinkMan.removeBlockPreDeleteFcn  PreDeleteFcn=Stateflow.SLINSF.SimulinkMan.unsafePredeleteFcn
  Handler : Subsystem
  Signal Conversion : SignalConversion
  SwitchForFreeSteering : Subsystem
  cmd : Outport  InitialOutput=[0 0]
  wires:
  Handler/1(cmd) -> Signal Conversion/1
  lightSignal/1 -> SwitchForFreeSteering/3(LightSens)
  SwitchForFreeSteering/1(Steering) -> Handler/1(steering)
  flagSteering/1 -> SwitchForFreeSteering/1(FlagSteering)
  PID/1 -> SwitchForFreeSteering/2(PID)
  fwd/1 -> Handler/2(fwd)
  Signal Conversion/1 -> cmd/1

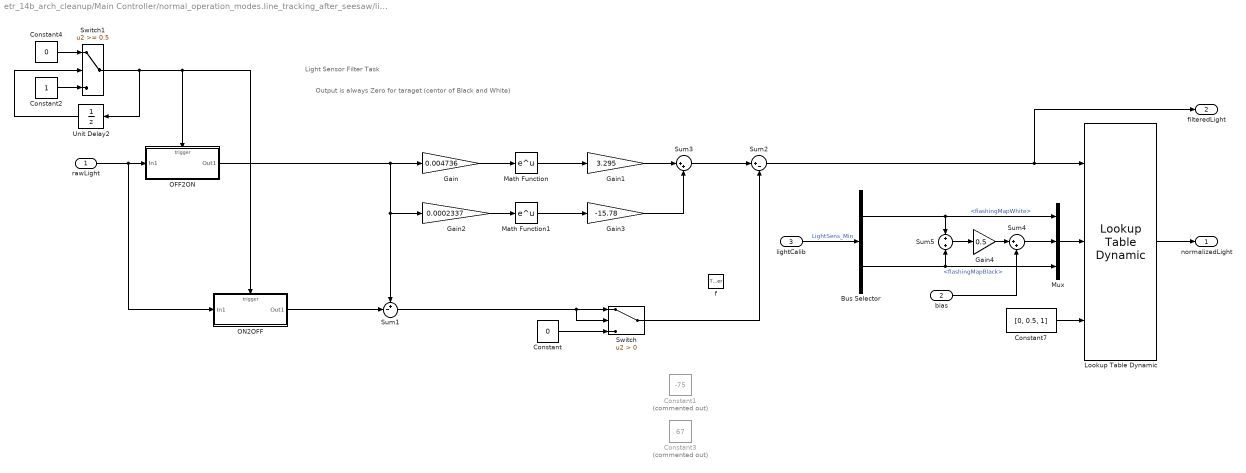
== system etr_14b_arch_cleanup/Main Controller/normal_operation_modes.line_tracking_after_seesaw/line_tracking_mode.Track.processLight ==
  note: Output is always Zero for taraget (centor of Black and White)
  note: Light Sensor Filter Task
  rawLight : Inport  OutDataTypeStr=single  PortDimensions=1
  bias : Inport  Port=2  OutDataTypeStr=single  PortDimensions=1
  lightCalib : Inport  Port=3  OutDataTypeStr=Bus: Light_Bus  PortDimensions=1
  f : TriggerPort  TriggerType=function-call
      settings: CopyFcn=Stateflow.SLINSF.SimulinkMan.removeBlockPreDeleteFcn  PreDeleteFcn=Stateflow.SLINSF.SimulinkMan.unsafePredeleteFcn
  Bus Selector : BusSelector  OutputSignals=flashingMapWhite,flashingMapBlack
  Constant : Constant  Value=0  OutDataTypeStr=single  SampleTime=-1
  Constant1 : Constant  Commented=on  Value=-75  OutDataTypeStr=single  SampleTime=-1
  Constant2 : Constant  OutDataTypeStr=uint8
  Constant3 : Constant  Commented=on  Value=67  OutDataTypeStr=single  SampleTime=-1
  Constant4 : Constant  Value=0  OutDataTypeStr=uint8
  Constant7 : Constant  Value=[0, 0.5, 1]  OutDataTypeStr=single  SampleTime=-1
  Gain : Gain  Gain=0.004736
  Gain1 : Gain  Gain=3.295
  Gain2 : Gain  Gain=0.0002337
  Gain3 : Gain  Gain=-15.78
  Gain4 : Gain  Gain=0.5
  Lookup Table Dynamic : simulink/Lookup Tables/Lookup Table Dynamic  LookUpMeth=Interpolation-Use End Values  OutDataTypeStr=fixdt('single')  OutputDataTypeScalingMode=Specify via dialog  OutDataType=fixdt('single')  OutScaling=[]  RndMeth=Simplest  DoSatur=off
  Math Function : Math  SaturateOnIntegerOverflow=on
  Math Function1 : Math  SaturateOnIntegerOverflow=on
  Mux : Mux  Inputs=3
  OFF2ON : Subsystem  TreatAsAtomicUnit=on
  ON2OFF : Subsystem  TreatAsAtomicUnit=on
  Sum1 : Sum  Inputs=+-|
  Sum2 : Sum  Inputs=|+-
  Sum3 : Sum  Inputs=|++
  Sum4 : Sum  Inputs=|++  OutDataTypeStr=single  RndMeth=Simplest
  Sum5 : Sum  Inputs=+|+
  Switch : Switch  Criteria=u2 > Threshold  RndMeth=Simplest
  Switch1 : Switch  Threshold=0.5
  Unit Delay2 : UnitDelay  SampleTime=-1
  normalizedLight : Outport  OutDataTypeStr=single  PortDimensions=1  InitialOutput=0
  filteredLight : Outport  Port=2  OutDataTypeStr=single  PortDimensions=1  InitialOutput=0
  wires:
  Bus Selector/2 -> Sum5/2, Mux/3  "<flashingMapBlack>"
  Mux/1 -> Lookup Table Dynamic/2
  Sum4/1 -> Mux/2
  bias/1 -> Sum4/2
  Constant7/1 -> Lookup Table Dynamic/3
  Lookup Table Dynamic/1 -> normalizedLight/1
  Sum2/1 -> filteredLight/1, Lookup Table Dynamic/1
  Switch/1 -> Sum2/2
  Sum3/1 -> Sum2/1
  Gain3/1 -> Sum3/2
  Gain1/1 -> Sum3/1
  Math Function1/1 -> Gain3/1
  Gain2/1 -> Math Function1/1
  Sum1/1 -> Switch/2, Switch/1
  Constant/1 -> Switch/3
  Math Function/1 -> Gain1/1
  Gain/1 -> Math Function/1
  OFF2ON/1(Out1) -> Gain2/1, Sum1/1, Gain/1
  ON2OFF/1(Out1) -> Sum1/2
  Unit Delay2/1 -> Switch1/2
  Constant4/1 -> Switch1/1
  Constant2/1 -> Switch1/3
  Switch1/1 -> Unit Delay2/1, OFF2ON/Trigger, ON2OFF/Trigger
  rawLight/1 -> ON2OFF/1(In1), OFF2ON/1(In1)
  Bus Selector/1 -> Mux/1, Sum5/1  "<flashingMapWhite>"
  Sum5/1 -> Gain4/1
  Gain4/1 -> Sum4/1
  lightCalib/1 -> Bus Selector/1  "LightSens_Min"

== system etr_14b_arch_cleanup/Main Controller/normal_operation_modes.line_tracking_after_seesaw/line_tracking_mode.balanceControl ==
  rawSensors : Inport  OutDataTypeStr=Bus: Sensors_Bus  PortDimensions=1
  lineTrackCmd : Inport  Port=2  OutDataTypeStr=single  PortDimensions=2
  f : TriggerPort  TriggerType=function-call
      settings: CopyFcn=Stateflow.SLINSF.SimulinkMan.removeBlockPreDeleteFcn  PreDeleteFcn=Stateflow.SLINSF.SimulinkMan.unsafePredeleteFcn
  Bus Selector : BusSelector  OutputSignals=gyro,theta_L,theta_R,battery
  Constant1 : Constant  Commented=on  Value=588  OutDataTypeStr=uint16
  Constant3 : Constant  Value=612  OutDataTypeStr=uint16
  Data Type Conversion2 : DataTypeConversion  OutDataTypeStr=single  RndMeth=Simplest
      settings: AttributesFormatString=Round = %<RndMeth>
  Demux : Demux  Outputs=2
  ForSimulation : Subsystem  TreatAsAtomicUnit=on  RTWFcnName=balance_control  RTWFileName=balancer
      settings: RTWFcnNameOpts=User specified  RTWFileNameOpts=User specified  FunctionWithSeparateData=on
  Low Pass Filter : Subsystem
  removeOffset : Subsystem
  leftPWM : Outport  OutDataTypeStr=single  PortDimensions=1
  rightPWM : Outport  Port=2
  wires:
  ForSimulation/1(pwm_l) -> rightPWM/1
  ForSimulation/2(pwm_r) -> leftPWM/1
  rawSensors/1 -> Bus Selector/1
  lineTrackCmd/1 -> Demux/1
  Constant3/1 -> Data Type Conversion2/1
  Data Type Conversion2/1 -> ForSimulation/4(gyro_offset)  "gyro_offset"
  Bus Selector/1 -> ForSimulation/3(gyro)  "<gyro>"
  Bus Selector/4 -> Low Pass Filter/1(u)  "<battery>"
  Low Pass Filter/1(y) -> ForSimulation/7(battery)
  Demux/1 -> ForSimulation/1(cmd_forward)
  Demux/2 -> ForSimulation/2(cmd_turn)
  Bus Selector/2 -> removeOffset/1(In1)  "<theta_L>"
  Bus Selector/3 -> removeOffset/2(In2)  "<theta_R>"
  removeOffset/1(Out1) -> ForSimulation/5(theta_m_l)
  removeOffset/2(Out2) -> ForSimulation/6(theta_m_r)

== system etr_14b_arch_cleanup/Main Controller/normal_operation_modes.line_tracking_after_seesaw/line_tracking_mode.phiController ==
  phi : Inport  OutDataTypeStr=single  PortDimensions=1
  desiredPhi : Inport  Port=2  OutDataTypeStr=single  PortDimensions=1
  battery : Inport  Port=3  OutDataTypeStr=double  PortDimensions=1
  f : TriggerPort  TriggerType=function-call
      settings: CopyFcn=Stateflow.SLINSF.SimulinkMan.removeBlockPreDeleteFcn  PreDeleteFcn=Stateflow.SLINSF.SimulinkMan.unsafePredeleteFcn
  Divide : Product  Inputs=*/
  Gain : Gain  Gain=-10
  Gain1 : Gain  Gain=100
  Saturation1 : Saturate  UpperLimit=100  LowerLimit=-100  OutDataTypeStr=single
  Sum : Sum  Inputs=|+-
  cmd : Outport
  wires:
  Saturation1/1 -> cmd/1
  Gain/1 -> Divide/1
  Divide/1 -> Gain1/1
  Gain1/1 -> Saturation1/1
  battery/1 -> Divide/2
  Sum/1 -> Gain/1
  phi/1 -> Sum/2
  desiredPhi/1 -> Sum/1

== system etr_14b_arch_cleanup/Main Controller/normal_operation_modes.line_tracking_after_seesaw/line_tracking_mode.turnLightOn ==
  f : TriggerPort  TriggerType=function-call
      settings: CopyFcn=Stateflow.SLINSF.SimulinkMan.removeBlockPreDeleteFcn  PreDeleteFcn=Stateflow.SLINSF.SimulinkMan.unsafePredeleteFcn
  Light Sensor Switch ON : S-Function  FunctionName=sfun_light_sw  Parameters=-1,ip,sw  EnableBusSupport=off  mask(Light Sensor ON/OFF Switch){ip=S3, sw=ON}
      mask prompts: ip "port:"; sw "switch"
      mask help: LEGO Mindstorms NXT Light Sensor switch.
      mask init:
      | [data, map]=imread('LIGHT_SENSOR.gif');
      | pic=ind2rgb(data,map);
      mask TypeOptions ip: S1 | S2 | S3 | S4
      mask TypeOptions sw: ON | OFF
      mask Display:
      | image(pic)
      | color('red')
      | fprintf('%s, %s',ip,sw)

== system etr_14b_arch_cleanup/Main Controller/normal_operation_modes.line_tracking_mode/line_tracking_mode.Speak ==
  f : TriggerPort  TriggerType=function-call
      settings: CopyFcn=Stateflow.SLINSF.SimulinkMan.removeBlockPreDeleteFcn  PreDeleteFcn=Stateflow.SLINSF.SimulinkMan.unsafePredeleteFcn
  Constant : Constant  Value=50
  Speaker : legonxtlib/Speaker  sinputMode=Volume only  sspeakerFreq=800  sspeakerVolume=50  sspeakerDuration=100
  wires:
  Constant/1 -> Speaker/1

== system etr_14b_arch_cleanup/Main Controller/normal_operation_modes.line_tracking_mode/line_tracking_mode.Track.analyzeEncoders ==
  rawSensors : Inport  OutDataTypeStr=Bus: Sensors_Bus  PortDimensions=1
  f : TriggerPort  TriggerType=function-call
      settings: CopyFcn=Stateflow.SLINSF.SimulinkMan.removeBlockPreDeleteFcn  PreDeleteFcn=Stateflow.SLINSF.SimulinkMan.unsafePredeleteFcn
  AngleCounter : Subsystem
  Bus Creator : BusCreator  Inputs=2
  Bus Selector : BusSelector  OutputSignals=theta_R,theta_L
  Signal Conversion : SignalConversion
  Signal Conversion1 : SignalConversion
  AngleCount : Outport  OutDataTypeStr=uint8  PortDimensions=1  InitialOutput=0
  EncoderReset : Outport  Port=2  OutDataTypeStr=single  PortDimensions=1  InitialOutput=0
  Angle : Outport  Port=3  OutDataTypeStr=single  PortDimensions=1  InitialOutput=0
  Distance : Outport  Port=4  OutDataTypeStr=single  PortDimensions=1  InitialOutput=0
  wires:
  rawSensors/1 -> Bus Selector/1
  Bus Creator/1 -> AngleCounter/1(EC)
  Bus Selector/1 -> Signal Conversion/1  "<theta_R>"
  Bus Selector/2 -> Signal Conversion1/1  "<theta_L>"
  Signal Conversion/1 -> Bus Creator/1  "R"
  Signal Conversion1/1 -> Bus Creator/2  "L"
  AngleCounter/1(AngleCount) -> AngleCount/1
  AngleCounter/2(EncoderReseted) -> EncoderReset/1
  AngleCounter/3(Angle) -> Angle/1
  AngleCounter/4(Distance) -> Distance/1

== system etr_14b_arch_cleanup/Main Controller/normal_operation_modes.line_tracking_mode/line_tracking_mode.Track.lineTracker ==
  lightSignal : Inport  OutDataTypeStr=single  PortDimensions=1
  flagSteering : Inport  Port=2  OutDataTypeStr=single  PortDimensions=1
  PID : Inport  Port=3  OutDataTypeStr=single  PortDimensions=5
  fwd : Inport  Port=4  OutDataTypeStr=single  PortDimensions=1
  f : TriggerPort  TriggerType=function-call
      settings: CopyFcn=Stateflow.SLINSF.SimulinkMan.removeBlockPreDeleteFcn  PreDeleteFcn=Stateflow.SLINSF.SimulinkMan.unsafePredeleteFcn
  Gain : Gain  Gain=100
  Handler : Subsystem
  LCD : legonxtlib/LCD  slcdStr=PID  slcdLine=6  slcdFormat=Decimal
  Signal Conversion : SignalConversion
  SwitchForFreeSteering : Subsystem
  cmd : Outport  InitialOutput=[0 0]
  wires:
  Handler/1(cmd) -> Signal Conversion/1
  lightSignal/1 -> SwitchForFreeSteering/3(LightSens)
  SwitchForFreeSteering/1(Steering) -> Gain/1, Handler/1(steering)
  flagSteering/1 -> SwitchForFreeSteering/1(FlagSteering)
  PID/1 -> SwitchForFreeSteering/2(PID)
  fwd/1 -> Handler/2(fwd)
  Signal Conversion/1 -> cmd/1
  Gain/1 -> LCD/1

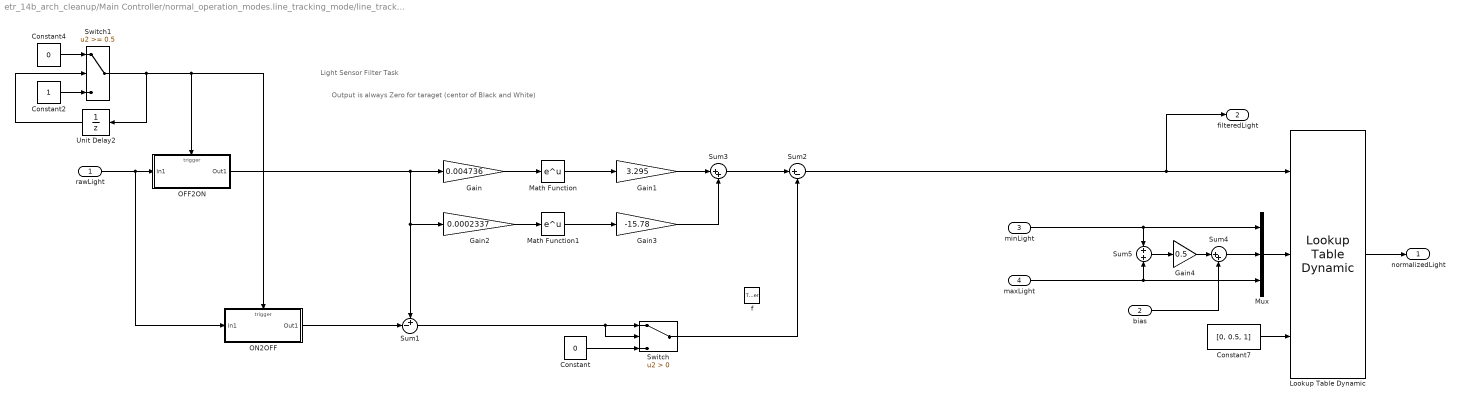
== system etr_14b_arch_cleanup/Main Controller/normal_operation_modes.line_tracking_mode/line_tracking_mode.Track.processLight ==
  note: Output is always Zero for taraget (centor of Black and White)
  note: Light Sensor Filter Task
  rawLight : Inport  OutDataTypeStr=single  PortDimensions=1
  bias : Inport  Port=2  OutDataTypeStr=single  PortDimensions=1
  minLight : Inport  Port=3  OutDataTypeStr=single  PortDimensions=1
  maxLight : Inport  Port=4  OutDataTypeStr=single  PortDimensions=1
  f : TriggerPort  TriggerType=function-call
      settings: CopyFcn=Stateflow.SLINSF.SimulinkMan.removeBlockPreDeleteFcn  PreDeleteFcn=Stateflow.SLINSF.SimulinkMan.unsafePredeleteFcn
  Constant : Constant  Value=0  OutDataTypeStr=single  SampleTime=-1
  Constant2 : Constant  OutDataTypeStr=uint8
  Constant4 : Constant  Value=0  OutDataTypeStr=uint8
  Constant7 : Constant  Value=[0, 0.5, 1]  OutDataTypeStr=single  SampleTime=-1
  Gain : Gain  Gain=0.004736
  Gain1 : Gain  Gain=3.295
  Gain2 : Gain  Gain=0.0002337
  Gain3 : Gain  Gain=-15.78
  Gain4 : Gain  Gain=0.5
  Lookup Table Dynamic : simulink/Lookup Tables/Lookup Table Dynamic  LookUpMeth=Interpolation-Use End Values  OutDataTypeStr=fixdt('single')  OutputDataTypeScalingMode=Specify via dialog  OutDataType=fixdt('single')  OutScaling=[]  RndMeth=Simplest  DoSatur=off
  Math Function : Math  SaturateOnIntegerOverflow=on
  Math Function1 : Math  SaturateOnIntegerOverflow=on
  Mux : Mux  Inputs=3
  OFF2ON : Subsystem  TreatAsAtomicUnit=on
  ON2OFF : Subsystem  TreatAsAtomicUnit=on
  Sum1 : Sum  Inputs=+-|
  Sum2 : Sum  Inputs=|+-
  Sum3 : Sum  Inputs=|++
  Sum4 : Sum  Inputs=|++  OutDataTypeStr=single  RndMeth=Simplest
  Sum5 : Sum  Inputs=+|+
  Switch : Switch  Criteria=u2 > Threshold  RndMeth=Simplest
  Switch1 : Switch  Threshold=0.5
  Unit Delay2 : UnitDelay  SampleTime=-1
  normalizedLight : Outport  OutDataTypeStr=single  PortDimensions=1  InitialOutput=0
  filteredLight : Outport  Port=2  OutDataTypeStr=single  PortDimensions=1  InitialOutput=0
  wires:
  minLight/1 -> Sum5/1, Mux/1
  Mux/1 -> Lookup Table Dynamic/2
  Sum4/1 -> Mux/2
  Sum5/1 -> Gain4/1
  bias/1 -> Sum4/2
  Constant7/1 -> Lookup Table Dynamic/3
  Lookup Table Dynamic/1 -> normalizedLight/1
  Sum2/1 -> filteredLight/1, Lookup Table Dynamic/1
  Switch/1 -> Sum2/2
  Sum3/1 -> Sum2/1
  Gain3/1 -> Sum3/2
  Gain1/1 -> Sum3/1
  Math Function1/1 -> Gain3/1
  Gain2/1 -> Math Function1/1
  Sum1/1 -> Switch/2, Switch/1
  Constant/1 -> Switch/3
  Math Function/1 -> Gain1/1
  Gain/1 -> Math Function/1
  OFF2ON/1(Out1) -> Gain2/1, Sum1/1, Gain/1
  ON2OFF/1(Out1) -> Sum1/2
  Unit Delay2/1 -> Switch1/2
  Constant4/1 -> Switch1/1
  Constant2/1 -> Switch1/3
  Switch1/1 -> Unit Delay2/1, OFF2ON/Trigger, ON2OFF/Trigger
  rawLight/1 -> ON2OFF/1(In1), OFF2ON/1(In1)
  Gain4/1 -> Sum4/1
  maxLight/1 -> Sum5/2, Mux/3

== system etr_14b_arch_cleanup/Main Controller/normal_operation_modes.line_tracking_mode/line_tracking_mode.balanceControl ==
  rawSensors : Inport  OutDataTypeStr=Bus: Sensors_Bus  PortDimensions=1
  lineTrackCmd : Inport  Port=2  OutDataTypeStr=single  PortDimensions=2
  gyroTrick : Inport  Port=3  OutDataTypeStr=single  PortDimensions=1
  f : TriggerPort  TriggerType=function-call
      settings: CopyFcn=Stateflow.SLINSF.SimulinkMan.removeBlockPreDeleteFcn  PreDeleteFcn=Stateflow.SLINSF.SimulinkMan.unsafePredeleteFcn
  Bus Selector : BusSelector  OutputSignals=gyro,theta_L,theta_R,battery
  Constant1 : Constant  Commented=on  Value=588  OutDataTypeStr=uint16
  Constant3 : Constant  Value=612  OutDataTypeStr=uint16
  Data Type Conversion2 : DataTypeConversion  OutDataTypeStr=single  RndMeth=Simplest
      settings: AttributesFormatString=Round = %<RndMeth>
  Demux : Demux  Outputs=2
  ForSimulation : Subsystem  TreatAsAtomicUnit=on  RTWFcnName=balance_control  RTWFileName=balancer
      settings: RTWFcnNameOpts=User specified  RTWFileNameOpts=User specified  FunctionWithSeparateData=on
  Low Pass Filter : Subsystem
  Sum : Sum
  leftPWM : Outport  OutDataTypeStr=single  PortDimensions=1
  rightPWM : Outport  Port=2
  wires:
  ForSimulation/1(pwm_l) -> rightPWM/1
  ForSimulation/2(pwm_r) -> leftPWM/1
  rawSensors/1 -> Bus Selector/1
  lineTrackCmd/1 -> Demux/1
  Bus Selector/2 -> ForSimulation/5(theta_m_l)  "<theta_L>"
  Bus Selector/3 -> ForSimulation/6(theta_m_r)  "<theta_R>"
  Bus Selector/1 -> ForSimulation/3(gyro)  "<gyro>"
  Bus Selector/4 -> Low Pass Filter/1(u)  "<battery>"
  Low Pass Filter/1(y) -> ForSimulation/7(battery)
  Demux/1 -> ForSimulation/1(cmd_forward)
  Demux/2 -> ForSimulation/2(cmd_turn)
  Constant3/1 -> Data Type Conversion2/1
  Data Type Conversion2/1 -> Sum/1  "gyro_offset"
  gyroTrick/1 -> Sum/2
  Sum/1 -> ForSimulation/4(gyro_offset)

== system etr_14b_arch_cleanup/Main Controller/normal_operation_modes.line_tracking_mode/line_tracking_mode.phiController ==
  phi : Inport  OutDataTypeStr=single  PortDimensions=1
  desiredPhi : Inport  Port=2  OutDataTypeStr=single  PortDimensions=1
  battery : Inport  Port=3  OutDataTypeStr=double  PortDimensions=1
  f : TriggerPort  TriggerType=function-call
      settings: CopyFcn=Stateflow.SLINSF.SimulinkMan.removeBlockPreDeleteFcn  PreDeleteFcn=Stateflow.SLINSF.SimulinkMan.unsafePredeleteFcn
  Divide : Product  Inputs=*/
  Gain : Gain  Gain=-10
  Gain1 : Gain  Gain=100
  Saturation1 : Saturate  UpperLimit=100  LowerLimit=-100  OutDataTypeStr=single
  Sum : Sum  Inputs=|+-
  cmd : Outport
  wires:
  Saturation1/1 -> cmd/1
  Gain/1 -> Divide/1
  Divide/1 -> Gain1/1
  Gain1/1 -> Saturation1/1
  battery/1 -> Divide/2
  Sum/1 -> Gain/1
  phi/1 -> Sum/2
  desiredPhi/1 -> Sum/1

== system etr_14b_arch_cleanup/Main Controller/normal_operation_modes.line_tracking_mode/line_tracking_mode.turnLightOn ==
  f : TriggerPort  TriggerType=function-call
      settings: CopyFcn=Stateflow.SLINSF.SimulinkMan.removeBlockPreDeleteFcn  PreDeleteFcn=Stateflow.SLINSF.SimulinkMan.unsafePredeleteFcn
  Light Sensor Switch ON : S-Function  FunctionName=sfun_light_sw  Parameters=-1,ip,sw  EnableBusSupport=off  mask(Light Sensor ON/OFF Switch){ip=S3, sw=ON}
      mask prompts: ip "port:"; sw "switch"
      mask help: LEGO Mindstorms NXT Light Sensor switch.
      mask init:
      | [data, map]=imread('LIGHT_SENSOR.gif');
      | pic=ind2rgb(data,map);
      mask TypeOptions ip: S1 | S2 | S3 | S4
      mask TypeOptions sw: ON | OFF
      mask Display:
      | image(pic)
      | color('red')
      | fprintf('%s, %s',ip,sw)
